simulink model "proceso_dblcart"  (R2014a)
settings: Solver=ode23  SolverMode=SingleTasking  StartTime=0  StopTime=3  MaxStep=0.1  RelTol=1e-3  AbsTol=1e-6
PostLoadFcn:
  | crtanim2([],[],[],0,1);
model workspace (MAT data in the model file):
  m1 = 936
  m2 = 473
  k1 = 44787
  k2 = 41032
  c1 = 13843
  c2 = 1273
libraries: simulink x3
Description:
  | Double Spring Mass System
  | 
  | This example shows how to model a double spring-mass-damper system with a periodically
  | varying forcing function.  Associated with the example is an animation function
  | that will automatically open a figure window and display to it. In this system,
  | the only sensor is attached to the mass on the left, and the actuator is
  | attached to the mass on the left. State estimation and LQR control are used.
settings Model: ExtModeAutoUpdateStatusClock=off  Creator=The MathWorks Inc.  LastModifiedBy=juancarlos
settings DataIOCC: ExternalInput=[]  InitialState=[]  LimitDataPoints=off  SaveOutput=off  SaveTime=off
settings OptimizationCC: BlockReduction=off  BooleanDataType=off  InitFltsAndDblsToZero=on  BufferReusableBoundary=off
settings DebuggingCC: SaveWithParameterizedLinksMsg=none  UnderspecifiedInitializationDetection=Classic  SignalResolutionControl=TryResolveAllWithWarning  SolverPrmCheckMsg=none  MultiTaskDSMMsg=warning  MultiTaskCondExecSysMsg=none  FcnCallInpInsideContextMsg=UseLocalSettings  BusObjectLabelMismatch=none
settings HardwareCC: TargetBitPerLong=64  TargetBitPerPointer=64  TargetLongLongMode=on  TargetIntDivRoundTo=Zero  TargetEndianess=LittleEndian  TargetWordSize=64  TargetHWDeviceType=MATLAB Host  ProdEqTarget=off
settings RTWCC: IncludeERTFirstTime=on
settings GRTTargetCC: TargetFcnLib=ansi_tfl_tmw.mat  CombineOutputUpdateFcns=off  GRTInterface=on

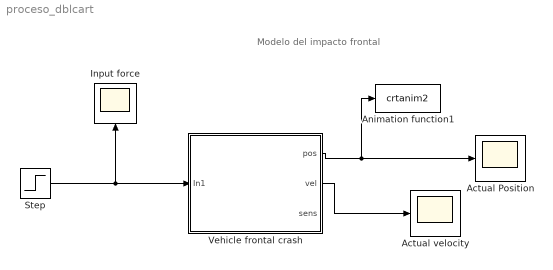
== system proceso_dblcart ==
  note: Modelo del impacto frontal
  Actual Position : Scope
      settings: TickLabels=on  TimeRange=3  YMin=-3  YMax=0
  Actual velocity : Scope
      settings: TickLabels=on  TimeRange=3  YMin=-9.5  YMax=1.5  SaveName=ScopeData2
  Animation function1 : S-Function  FunctionName=crtanim2  Parameters=0.1  EnableBusSupport=off
      settings: DeleteFcn=shh = get(0,'ShowHiddenHandles');set(0,'ShowHiddenHandles','on');if ~isempty(findobj('type','figure','name','dblcart1 Animation'));close('dblcart1 Animation'); end;set(0,'ShowHiddenHandles',shh);
  Input force : Scope
      settings: YMin=-50000  YMax=50000
  Step : Step  Time=0  After=40000  SampleTime=.2
  Vehicle frontal crash : Subsystem
      mask Display: image(imread('Captura89','png'));
  wires:
  Vehicle frontal crash/1(pos) -> Animation function1/1, Actual Position/1
  Step/1 -> Input force/1, Vehicle frontal crash/1(In1)
  Vehicle frontal crash/2(vel) -> Actual velocity/1

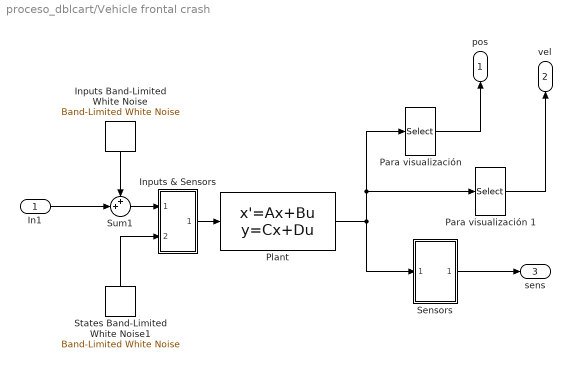
== system proceso_dblcart/Vehicle frontal crash ==
  In1 : Inport
  Inputs Band-Limited White Noise : simulink/Sources/Band-Limited White Noise  Cov=[1000]  Ts=0.05  seed=[23341]
  Inputs & Sensors : Subsystem
  "Para visualización " : Selector  InputPortWidth=4  Indices=[1,3]
  Para visualización 1 : Selector  InputPortWidth=4  Indices=[2,4]
  Plant : StateSpace  A=[0 1 0 0; -(k1+k2)/m1 -(c1+c2)/m1 k2/m1 c2/m1; 0 0 0 1;k2/m2 c2/m2 -k2/m2 -c2/m2]  B=[0 .1; -1/m1 1; 0 .1; -1/m2 0]  C=[1 0 0 0;0 1 0 0;0 0 1 0; 0 0 0 1]  D=[0 0;0 0;0 0; 0 0]  X0=[0 ;0 ; 0; 0]
  Sensors : Subsystem
  States Band-Limited White Noise1 : simulink/Sources/Band-Limited White Noise  Cov=[0.01]  Ts=0.01  seed=[23341]
  Sum1 : Sum  Inputs=++|  SaturateOnIntegerOverflow=on  InputSameDT=on  OutDataTypeStr=Inherit: Same as first input
  pos : Outport
  vel : Outport  Port=2
  sens : Outport  Port=3
  wires:
  In1/1 -> Sum1/2
  Plant/1 -> Sensors/1(In1), "Para visualización "/1, Para visualización 1/1
  Sum1/1 -> Inputs & Sensors/1(In1)
  Inputs Band-Limited White Noise/1 -> Sum1/1
  "Para visualización "/1 -> pos/1
  Sensors/1(Out1) -> sens/1
  States Band-Limited White Noise1/1 -> Inputs & Sensors/2(In2)
  Inputs & Sensors/1(Out1) -> Plant/1
  Para visualización 1/1 -> vel/1

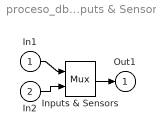
== system proceso_dblcart/Vehicle frontal crash/Inputs & Sensors ==
  In1 : Inport
  In2 : Inport  Port=2
  Inputs & Sensors : Mux  Inputs=2
  Out1 : Outport  InitialOutput=0
  wires:
  In1/1 -> Inputs & Sensors/1
  In2/1 -> Inputs & Sensors/2
  Inputs & Sensors/1 -> Out1/1

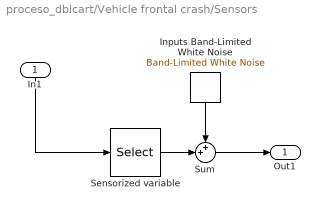
== system proceso_dblcart/Vehicle frontal crash/Sensors ==
  In1 : Inport
  Inputs Band-Limited White Noise : simulink/Sources/Band-Limited White Noise  Cov=[2000]  Ts=0.1  seed=[23341]
  Sensorized variable : Selector  InputPortWidth=4  Indices=3
  Sum : Sum  Inputs=++|
  Out1 : Outport
  wires:
  Sensorized variable/1 -> Sum/2
  In1/1 -> Sensorized variable/1
  Inputs Band-Limited White Noise/1 -> Sum/1
  Sum/1 -> Out1/1
